simulink model "candyDetectionModel"  (R2023a)
settings: Solver=VariableStepAuto  StartTime=0.0  StopTime=2  RelTol=1e-3
undefined symbols (not defined in the file or in its folder): gray
libraries: visionsources x1, visiongeotforms x1
settings Model: Creator=Rohanlal Das  LastModifiedBy=Rohanlal Das

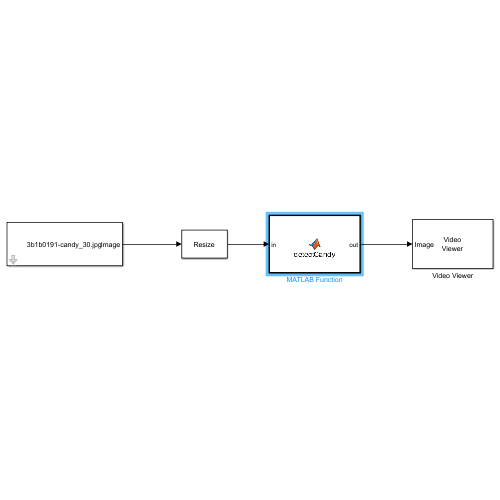
[thumbnail: Simulink's stored preview of the top-level diagram]
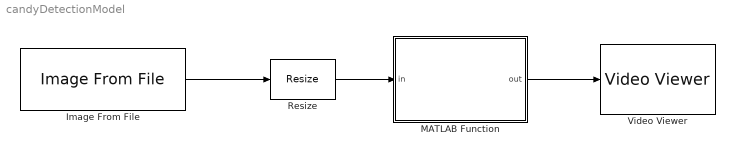
== system candyDetectionModel ==
  Image From File : visionsources/Image From File  Tag=vipblks_nd  FileName=C:\yolo\candyimages\images\3b1b0191-candy_30.jpg  Ts=inf  imagePorts=One multidimensional signal  OutPortLabels=R|G|B  ImageDataType=uint8  sdImageDataType=uint(8)  Signed=on  WordLength=16  FractionLengthMode=User-defined  FractionLength=15
  MATLAB Function : MATLAB Function  TreatAsAtomicUnit=on
  Resize : visiongeotforms/Resize  specify=Output size as a percentage of input size  rfactor=[320 320]  outCols=25  outRows=25  outRowsCols=[25 35]  interp_method=Nearest neighbor  antialias=on  useROI=off  roiFlag=off  roundingMode=Nearest  overflowMode=on  prodOutputMode=Binary point scaling  prodOutputWordLength=32  prodOutputFracLength=10
  Video Viewer : VideoViewer  colormapValue=gray(256)  FigPos=[266.6 779.6 950.4 613.6]
  wires:
  Image From File/1 -> Resize/1
  Resize/1 -> MATLAB Function/1(in)
  MATLAB Function/1(out) -> Video Viewer/1

== matlab function candyDetectionModel/MATLAB Function ==
  data: in input; out output
function out = detectCandy(in)
%#codegen

% Declare functions that are not supported for code generation
coder.extrinsic('evalin', 'detect', 'insertObjectAnnotation', ...
                'cellstr', 'string', 'strcat');

% Preinitialize output to match input image
out = in;

% Load detector from base workspace
detector = evalin('base', 'detector');

% Run detection using GPU
[bboxes, scores, labels] = detect(detector, in, 'ExecutionEnvironment', 'gpu');

% Annotate detections (if any)
if ~isempty(bboxes)
    labelStr = strcat(cellstr(labels), " ", string(round(scores * 100)), "%");
    out = insertObjectAnnotation(in, "rectangle", bboxes, labelStr, ...
        'FontSize', 22, 'LineWidth', 6, 'TextBoxOpacity', 0.8);
end
